simulink model "Tasks_union_3"  (R2020b)
settings: Solver=FixedStepAuto  StartTime=0.0  StopTime=11  FixedStep=0.001  RelTol=1e-3
values from neighbouring files (symbols this model uses):
  a = evalin('base','a')    [Coriolis.m]    (also in init.m = 0.5)
  a0 = 0.99    [init.m]
  ac = mass_can*(l1*l2)    (= 0.5)    [init.m]
  berta = 0.98    [init.m]
  csi = 1    [init.m]
  e_max = 0.01    [init.m]
  F_int_max = [2;2]    [init.m]
  F_max = [2;2]    [init.m]
  g = 9.81    [init.m]
  I1 = evalin('base','I1')    [Mass.m]    (also in init.m = 1)
  I2 = evalin('base','I2')    [Mass.m]    (also in init.m = 1)
  Ic = mass_can*l2^2    (= 0.5)    [init.m]
  k_can = 500    [init.m]
  k_shelf = k_table    (= 10000)    [init.m]
  k_table = 10000    [init.m]
  k_wall = k_table    (= 10000)    [init.m]
  l1 = evalin('base','l1')    [Jacobianoa.m]    (also in Mass.m; cin_dir.m; init.m = 1)
  l2 = evalin('base','l2')    [Jacobianoa.m]    (also in Mass.m; cin_dir.m; init.m = 1)
  l_can = 0.1    [init.m]
  M = 0.1    [init.m]
  m1 = evalin('base','m1')    [Mass.m]    (also in init.m = 1)
  m2 = evalin('base','m2')    [Mass.m]    (also in init.m = 1)
  mass = 0.1    [init.m]
  mass_can = 0.5    [init.m]
  x_can = 0.5    [init.m]
  x_wall = 1.5    [init.m]
  y_shelf = 0.5    [init.m]
  y_table = 0    [init.m]
libraries: simulink x3
settings Model: Creator=chiara-s  LastModifiedBy=giorg

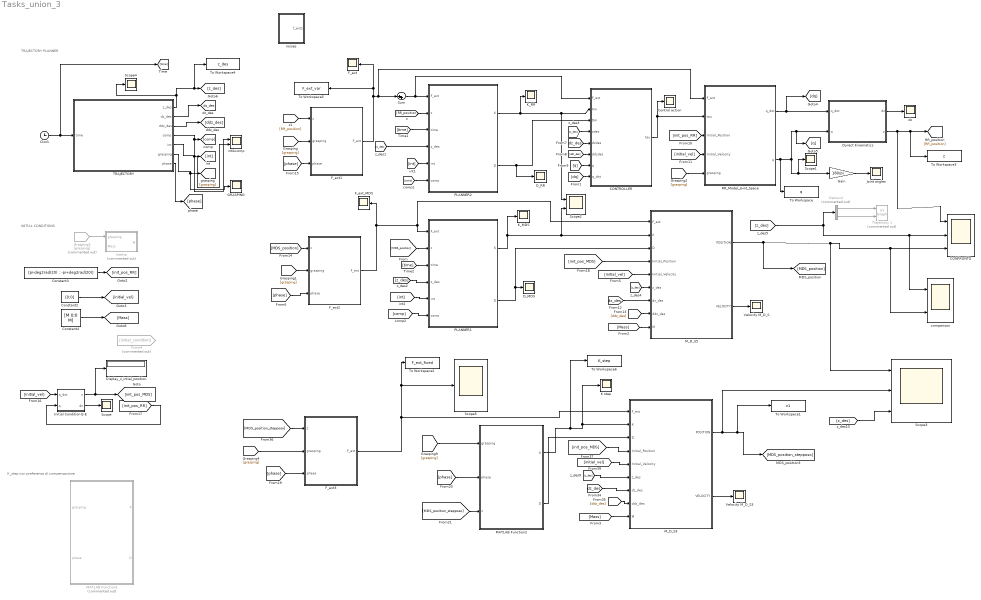
== system Tasks_union_3 ==
  note: K_step con preferenza di compensazione
  note: INITIAL CONDITIONS
  note: TRAJECTORY PLANNER
  CONFRONTO : Scope  NumInputPorts=3
  CONTROLLER : MATLAB Function  TreatAsAtomicUnit=on
  Clock : Clock
  Constant2 : Constant  Value=[0;0]
  Constant3 : Constant  Value=[pi-deg2rad(20) ; -pi+deg2rad(20)]  VectorParams1D=off
  Constant4 : Constant  Value=[M 0;0 M]
  Control action : Scope
  D_MDS : Scope
  D_RR : Scope
  Demux2 : Demux  Commented=on  Outputs=2
  Display_z_intial_position : Display
  Dyrect Kinematics : MATLAB Function  TreatAsAtomicUnit=on
  F_ext : Scope
  F_ext1 : MATLAB Function  TreatAsAtomicUnit=on
  F_ext2 : MATLAB Function  TreatAsAtomicUnit=on
  F_ext3 : MATLAB Function  TreatAsAtomicUnit=on
  F_ext_MDS : Scope
  From4 : From  Commented=on  GotoTag=initial_condition
  GRASPING : Scope
  Gain : Gain  Gain=180/pi
  Grasping3 : From  Commented=on  GotoTag=grasping
  "Inertia " : MATLAB Function  Commented=on  TreatAsAtomicUnit=on
  Initial Condition E-E : MATLAB Function  TreatAsAtomicUnit=on
  Joint angles : Scope
  K step : Scope
  K_MDS : Scope
  K_RR : Scope
  MATLAB Function1 : MATLAB Function  Commented=on  TreatAsAtomicUnit=on
  MATLAB Function2 : MATLAB Function  TreatAsAtomicUnit=on
  M_D_S3 : Subsystem
  M_D_S5 : Subsystem
  PLANNER1 : Subsystem
  PLANNER2 : Subsystem
  RR_Model_Joint_Space : Subsystem
  Scope{,1,4..5} (4 alike) : Scope
  Scope2 : Scope  NumInputPorts=2
  Scope3 : Scope  NumInputPorts=3
  Sum : Sum  Inputs=|++
  TRAJECTORY : Subsystem
  To Workspace : ToWorkspace  VariableName=q  SaveFormat=Timeseries  SampleTime=-1
  To Workspace1 : ToWorkspace  VariableName=z1  SaveFormat=Timeseries  SampleTime=-1
  To Workspace2 : ToWorkspace  VariableName=F_ext_fixed  SaveFormat=Timeseries  SampleTime=-1
  To Workspace3 : ToWorkspace  VariableName=z  SaveFormat=Timeseries  SampleTime=-1
  To Workspace4 : ToWorkspace  VariableName=z_des  SaveFormat=Timeseries  SampleTime=-1
      settings: Save2DSignal=2-D array (concatenate along first dimension)
  To Workspace5 : ToWorkspace  VariableName=F_ext_var  SaveFormat=Timeseries  SampleTime=-1
  To Workspace6 : ToWorkspace  VariableName=K_step  SaveFormat=Timeseries  SampleTime=-1
  Trajectory 1 : simulink/Sinks/XY Graph  Commented=on  xmin=-2  xmax=2  ymin=-2  ymax=2  st=-1
  Velocity M_D_S : Scope
  Velocity M_D_S3 : Scope
  comparison : Scope  NumInputPorts=2
  dz : Scope
  int&comp : Scope  NumInputPorts=2
  noises : Subsystem
  tag scope: dz_des=global
  wires:
  TRAJECTORY/4(comp) -> int&comp/1, [comp]
  [grasping] -> RR_Model_Joint_Space/5(grasping)
  [q] -> CONTROLLER/7(q)
  M_D_S5/1(POSITION) -> [MDS_position], Scope3/1, comparison/2, CONFRONTO/3
  Demux2/1 -> Trajectory 1/1
  M_D_S5/2(VELOCITY) -> Velocity M_D_S/1
  [dz_des] -> CONTROLLER/5(dzdes)
  Initial Condition E-E/2(dz) -> Scope/1
  [ddz_des] -> M_D_S5/8(ddz_des)
  [z_des] -> CONFRONTO/2, comparison/1, Demux2/1
  [grasping] -> F_ext1/2(grasping)
  [initial_vel] -> M_D_S5/5(Initial_Velocity)
  CONTROLLER/1(tau) -> Control action/1, RR_Model_Joint_Space/2(tau)
  [init_pos_RR] -> RR_Model_Joint_Space/3(Initial_Position)
  Gain/1 -> Joint angles/1
  [initial_vel] -> Initial Condition E-E/1(q_dot)
  TRAJECTORY/3(ddz_des) -> [ddz_des]
  RR_Model_Joint_Space/1(q_dot) -> [dq], Dyrect Kinematics/1(q_dot)
  Dyrect Kinematics/1(dz) -> dz/1
  TRAJECTORY/2(dz_des) -> [dz_des]
  Constant4/1 -> [Mass]
  TRAJECTORY/1(z_des) -> [z_des], To Workspace4/1, Scope4/1
  Initial Condition E-E/1(z) -> Display_z_intial_position/1, [init_pos_MDS]
  Constant3/1 -> [init_pos_RR]
  [dz_des] -> M_D_S5/7(dz_des)
  [ddz_des] -> CONTROLLER/6(ddzdes)
  [initial_vel] -> RR_Model_Joint_Space/4(Initial_Velocity)
  F_ext2/1(F_ext) -> PLANNER1/1(F_ext), M_D_S5/1(F_ext), F_ext_MDS/1
  Constant2/1 -> [initial_vel]
  [z_des] -> CONTROLLER/4(zdes)
  TRAJECTORY/6(grasping) -> [grasping], GRASPING/1
  [MDS_position] -> F_ext2/1(z)
  [RR_position] -> F_ext1/1(z)
  Dyrect Kinematics/2(z) -> CONFRONTO/1, To Workspace3/1, [RR_position]
  [grasping] -> F_ext2/2(grasping)
  [z_des] -> M_D_S5/6(z_des)
  Clock/1 -> TRAJECTORY/1(time), [time]
  RR_Model_Joint_Space/2(q) -> To Workspace/1, Scope1/1, Gain/1, Dyrect Kinematics/2(q), [q]
  Grasping3/1 -> "Inertia "/1(grasping)
  [dq] -> CONTROLLER/8(q_dot)
  [init_pos_RR] -> Initial Condition E-E/2(q)
  [Mass] -> M_D_S5/9(M)
  Demux2/2 -> Trajectory 1/2
  TRAJECTORY/5(int) -> int&comp/2, [int]
  TRAJECTORY/7(phase) -> [phase]
  [phase] -> F_ext2/3(phase)
  PLANNER1/1(K) -> K_MDS/1, Scope2/2, M_D_S5/2(K)
  PLANNER1/2(D) -> M_D_S5/3(D), D_MDS/1
  [MDS_position] -> PLANNER1/2(z)
  [time] -> PLANNER1/3(time)
  [z_des] -> PLANNER1/4(z_des)
  [int] -> PLANNER1/5(int)
  [comp] -> PLANNER1/6(comp)
  [phase] -> F_ext1/3(phase)
  F_ext1/1(F_ext) -> RR_Model_Joint_Space/1(F_ext), Sum/1, F_ext/1, To Workspace5/1
  [RR_position] -> PLANNER2/2(z)
  [time] -> PLANNER2/3(time)
  [z_des] -> PLANNER2/4(z_des)
  [comp] -> PLANNER2/6(comp)
  [int] -> PLANNER2/5(int)
  PLANNER2/1(K) -> K_RR/1, Scope2/1, CONTROLLER/2(Km)
  PLANNER2/2(D) -> D_RR/1, CONTROLLER/3(Dm)
  [init_pos_MDS] -> M_D_S5/4(Initial_Position)
  [initial_vel] -> M_D_S3/5(Initial_Velocity)
  MATLAB Function2/2(D) -> M_D_S3/3(D)
  MATLAB Function2/1(K) -> To Workspace6/1, K step/1, M_D_S3/2(K)
  [grasping] -> MATLAB Function2/1(grasping)
  M_D_S3/1(POSITION) -> Scope3/2, To Workspace1/1, [MDS_position_stepposo]
  [init_pos_MDS] -> M_D_S3/4(Initial_Position)
  M_D_S3/2(VELOCITY) -> Velocity M_D_S3/1
  [dz_des] -> M_D_S3/7(dz_des)
  [ddz_des] -> M_D_S3/8(ddz_des)
  [z_des] -> M_D_S3/6(z_des)
  [Mass] -> M_D_S3/9(M)
  [MDS_position_stepposo] -> F_ext3/1(z)
  [grasping] -> F_ext3/2(grasping)
  [phase] -> F_ext3/3(phase)
  F_ext3/1(F_ext) -> M_D_S3/1(F_ext), To Workspace2/1, Scope5/1
  [z_des] -> Scope3/3
  [phase] -> MATLAB Function2/2(phase)
  [MDS_position_stepposo] -> MATLAB Function2/3(z)
  Sum/1 -> CONTROLLER/1(F_ext), PLANNER2/1(F_ext)
  ? -> Sum/2

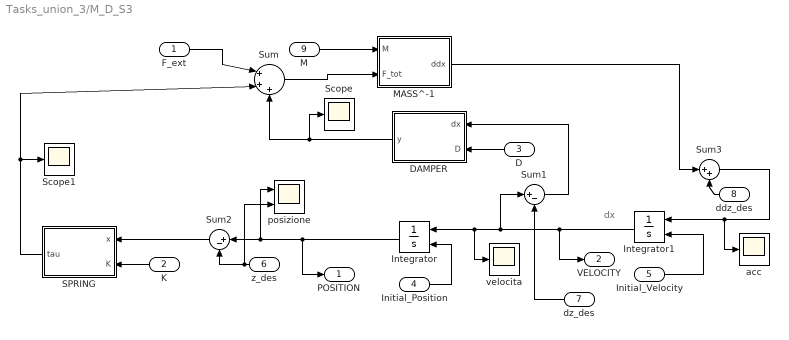
== system Tasks_union_3/M_D_S3 ==
  note: dx
  F_ext : Inport
  K : Inport  Port=2
  D : Inport  Port=3
  Initial_Position : Inport  Port=4
  Initial_Velocity : Inport  Port=5
  z_des : Inport  Port=6
  dz_des : Inport  Port=7
  ddz_des : Inport  Port=8
  M : Inport  Port=9
  DAMPER : MATLAB Function  TreatAsAtomicUnit=on
  Integrator : Integrator  InitialConditionSource=external
  Integrator1 : Integrator  InitialConditionSource=external
  MASS^-1 : MATLAB Function  TreatAsAtomicUnit=on
  SPRING : MATLAB Function  TreatAsAtomicUnit=on
  Scope : Scope
  Scope1 : Scope
  Sum : Sum  Inputs=|+++
  Sum1 : Sum  Inputs=|+-
  Sum2 : Sum  Inputs=|+-
  Sum3 : Sum  Inputs=|++
  acc : Scope
  posizione : Scope  NumInputPorts=2
  velocita : Scope
  POSITION : Outport
  VELOCITY : Outport  Port=2
  wires:
  Integrator1/1 -> velocita/1, Integrator/1, Sum1/1, VELOCITY/1
  SPRING/1(tau) -> Sum/2, Scope1/1
  Integrator/1 -> posizione/1, Sum2/1, POSITION/1
  DAMPER/1(y) -> Scope/1, Sum/3
  Sum/1 -> MASS^-1/2(F_tot)
  M/1 -> MASS^-1/1(M)
  D/1 -> DAMPER/2(D)
  K/1 -> SPRING/2(K)
  Initial_Velocity/1 -> Integrator1/2
  Initial_Position/1 -> Integrator/2
  z_des/1 -> posizione/2, Sum2/2
  Sum2/1 -> SPRING/1(x)
  MASS^-1/1(ddx) -> Sum3/1
  Sum1/1 -> DAMPER/1(dx)
  Sum3/1 -> acc/1, Integrator1/1
  dz_des/1 -> Sum1/2
  ddz_des/1 -> Sum3/2
  F_ext/1 -> Sum/1

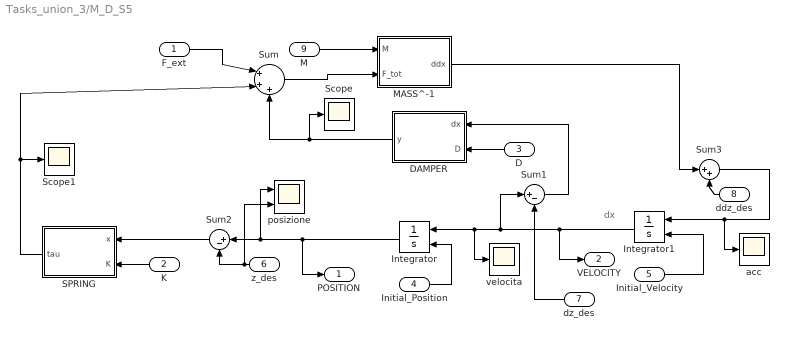
== system Tasks_union_3/M_D_S5 ==
  note: dx
  F_ext : Inport
  K : Inport  Port=2
  D : Inport  Port=3
  Initial_Position : Inport  Port=4
  Initial_Velocity : Inport  Port=5
  z_des : Inport  Port=6
  dz_des : Inport  Port=7
  ddz_des : Inport  Port=8
  M : Inport  Port=9
  DAMPER : MATLAB Function  TreatAsAtomicUnit=on
  Integrator : Integrator  InitialConditionSource=external
  Integrator1 : Integrator  InitialConditionSource=external
  MASS^-1 : MATLAB Function  TreatAsAtomicUnit=on
  SPRING : MATLAB Function  TreatAsAtomicUnit=on
  Scope : Scope
  Scope1 : Scope
  Sum : Sum  Inputs=|+++
  Sum1 : Sum  Inputs=|+-
  Sum2 : Sum  Inputs=|+-
  Sum3 : Sum  Inputs=|++
  acc : Scope
  posizione : Scope  NumInputPorts=2
  velocita : Scope
  POSITION : Outport
  VELOCITY : Outport  Port=2
  wires:
  Integrator1/1 -> velocita/1, Integrator/1, Sum1/1, VELOCITY/1
  SPRING/1(tau) -> Sum/2, Scope1/1
  Integrator/1 -> posizione/1, Sum2/1, POSITION/1
  DAMPER/1(y) -> Scope/1, Sum/3
  Sum/1 -> MASS^-1/2(F_tot)
  M/1 -> MASS^-1/1(M)
  D/1 -> DAMPER/2(D)
  K/1 -> SPRING/2(K)
  Initial_Velocity/1 -> Integrator1/2
  Initial_Position/1 -> Integrator/2
  z_des/1 -> posizione/2, Sum2/2
  Sum2/1 -> SPRING/1(x)
  MASS^-1/1(ddx) -> Sum3/1
  Sum1/1 -> DAMPER/1(dx)
  Sum3/1 -> acc/1, Integrator1/1
  dz_des/1 -> Sum1/2
  ddz_des/1 -> Sum3/2
  F_ext/1 -> Sum/1

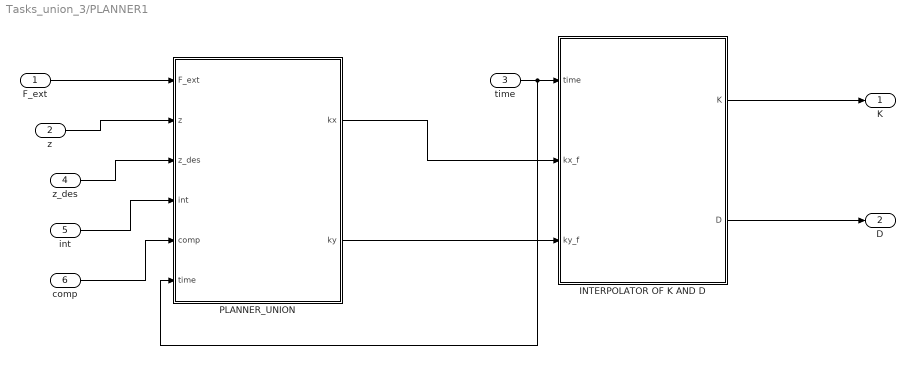
== system Tasks_union_3/PLANNER1 ==
  F_ext : Inport
  z : Inport  Port=2
  time : Inport  Port=3
  z_des : Inport  Port=4
  int : Inport  Port=5
  comp : Inport  Port=6
  "INTERPOLATOR OF K AND D " : MATLAB Function  TreatAsAtomicUnit=on
  PLANNER_UNION : MATLAB Function  TreatAsAtomicUnit=on
  K : Outport
  D : Outport  Port=2
  wires:
  time/1 -> "INTERPOLATOR OF K AND D "/1(time), PLANNER_UNION/6(time)
  "INTERPOLATOR OF K AND D "/2(D) -> D/1
  "INTERPOLATOR OF K AND D "/1(K) -> K/1
  PLANNER_UNION/2(ky) -> "INTERPOLATOR OF K AND D "/3(ky_f)
  PLANNER_UNION/1(kx) -> "INTERPOLATOR OF K AND D "/2(kx_f)
  int/1 -> PLANNER_UNION/4(int)
  comp/1 -> PLANNER_UNION/5(comp)
  F_ext/1 -> PLANNER_UNION/1(F_ext)
  z/1 -> PLANNER_UNION/2(z)
  z_des/1 -> PLANNER_UNION/3(z_des)

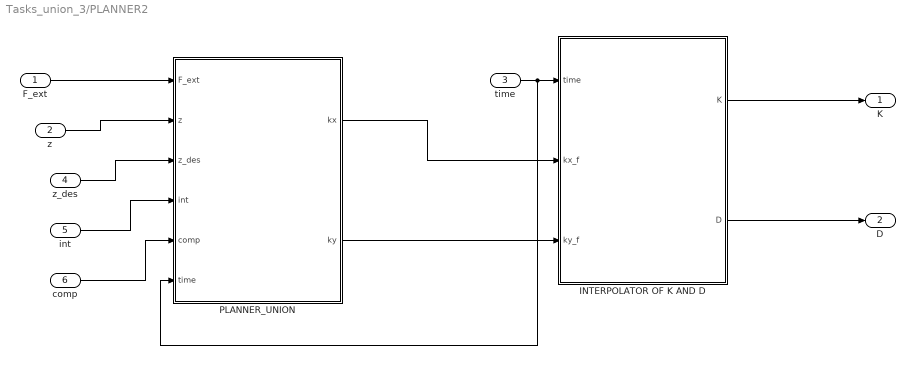
== system Tasks_union_3/PLANNER2 ==
  F_ext : Inport
  z : Inport  Port=2
  time : Inport  Port=3
  z_des : Inport  Port=4
  int : Inport  Port=5
  comp : Inport  Port=6
  "INTERPOLATOR OF K AND D " : MATLAB Function  TreatAsAtomicUnit=on
  PLANNER_UNION : MATLAB Function  TreatAsAtomicUnit=on
  K : Outport
  D : Outport  Port=2
  wires:
  time/1 -> "INTERPOLATOR OF K AND D "/1(time), PLANNER_UNION/6(time)
  "INTERPOLATOR OF K AND D "/2(D) -> D/1
  "INTERPOLATOR OF K AND D "/1(K) -> K/1
  PLANNER_UNION/2(ky) -> "INTERPOLATOR OF K AND D "/3(ky_f)
  PLANNER_UNION/1(kx) -> "INTERPOLATOR OF K AND D "/2(kx_f)
  int/1 -> PLANNER_UNION/4(int)
  comp/1 -> PLANNER_UNION/5(comp)
  F_ext/1 -> PLANNER_UNION/1(F_ext)
  z/1 -> PLANNER_UNION/2(z)
  z_des/1 -> PLANNER_UNION/3(z_des)

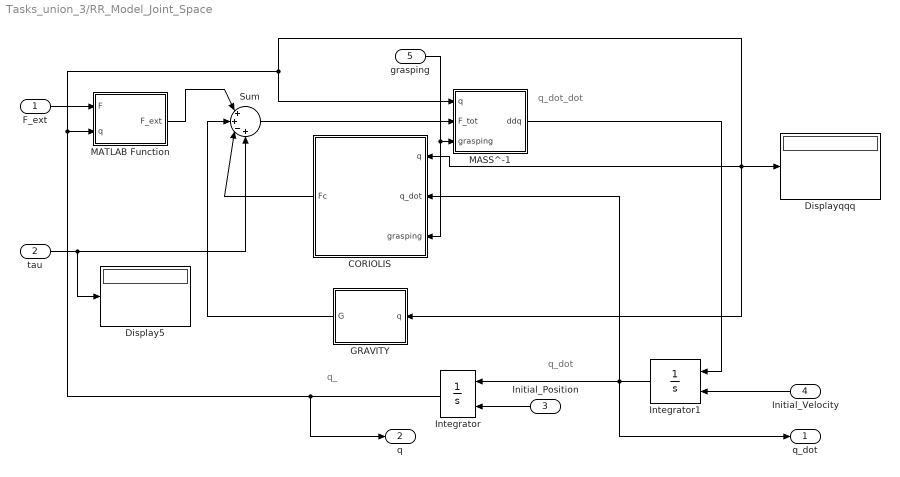
== system Tasks_union_3/RR_Model_Joint_Space ==
  note: q_dot
  note: q_dot_dot
  note: q_
  F_ext : Inport
  tau : Inport  Port=2
  Initial_Position : Inport  Port=3
  Initial_Velocity : Inport  Port=4
  grasping : Inport  Port=5
  CORIOLIS : MATLAB Function  TreatAsAtomicUnit=on
  Display5 : Display
  Displayqqq : Display
  GRAVITY : MATLAB Function  TreatAsAtomicUnit=on
  Integrator : Integrator  InitialConditionSource=external
  Integrator1 : Integrator  InitialConditionSource=external  InitialCondition=[0;0]
  MASS^-1 : MATLAB Function  TreatAsAtomicUnit=on
  MATLAB Function : MATLAB Function  TreatAsAtomicUnit=on
  Sum : Sum  Inputs=|++-+
  q_dot : Outport
  q : Outport  Port=2
  wires:
  GRAVITY/1(G) -> Sum/2
  MATLAB Function/1(F_ext) -> Sum/1
  Initial_Position/1 -> Integrator/2
  F_ext/1 -> MATLAB Function/1(F)
  Integrator/1 -> MASS^-1/1(q), GRAVITY/1(q), Displayqqq/1, CORIOLIS/1(q), MATLAB Function/2(q), q/1
  Integrator1/1 -> q_dot/1, CORIOLIS/2(q_dot), Integrator/1
  Initial_Velocity/1 -> Integrator1/2
  MASS^-1/1(ddq) -> Integrator1/1
  Sum/1 -> MASS^-1/2(F_tot)
  CORIOLIS/1(Fc) -> Sum/3
  tau/1 -> Display5/1, Sum/4
  grasping/1 -> CORIOLIS/3(grasping), MASS^-1/3(grasping)

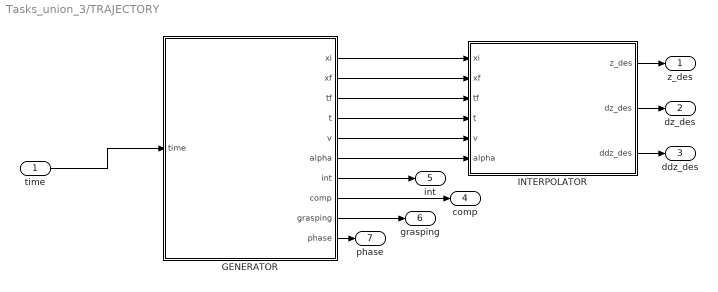
== system Tasks_union_3/TRAJECTORY ==
  time : Inport
  GENERATOR : MATLAB Function  TreatAsAtomicUnit=on
  INTERPOLATOR : MATLAB Function  TreatAsAtomicUnit=on
  z_des : Outport
  dz_des : Outport  Port=2
  ddz_des : Outport  Port=3
  comp : Outport  Port=4
  int : Outport  Port=5
  grasping : Outport  Port=6
  phase : Outport  Port=7
  wires:
  GENERATOR/1(xi) -> INTERPOLATOR/1(xi)
  GENERATOR/2(xf) -> INTERPOLATOR/2(xf)
  GENERATOR/3(tf) -> INTERPOLATOR/3(tf)
  GENERATOR/4(t) -> INTERPOLATOR/4(t)
  GENERATOR/5(v) -> INTERPOLATOR/5(v)
  GENERATOR/6(alpha) -> INTERPOLATOR/6(alpha)
  INTERPOLATOR/1(z_des) -> z_des/1
  INTERPOLATOR/2(dz_des) -> dz_des/1
  INTERPOLATOR/3(ddz_des) -> ddz_des/1
  GENERATOR/7(int) -> int/1
  GENERATOR/8(comp) -> comp/1
  GENERATOR/9(grasping) -> grasping/1
  GENERATOR/10(phase) -> phase/1
  time/1 -> GENERATOR/1(time)

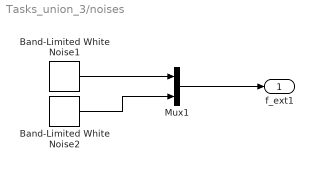
== system Tasks_union_3/noises ==
  Band-Limited White Noise1 : simulink/Sources/Band-Limited White Noise  Cov=0.0001  Ts=0.001  seed=[randi(10000,1)]
  Band-Limited White Noise2 : simulink/Sources/Band-Limited White Noise  Cov=0.0001  Ts=0.001  seed=[randi(10000,1)]
  Mux1 : Mux  Inputs=2
  f_ext1 : Outport
  wires:
  Band-Limited White Noise2/1 -> Mux1/2
  Band-Limited White Noise1/1 -> Mux1/1
  Mux1/1 -> f_ext1/1

== matlab function Tasks_union_3/Dyrect Kinematics ==
  data: q_dot input double size=2; dz output double size=2; q input double size=2; z output double size=2; l1 parameter; l2 parameter
function [dz,z] = fcn(q_dot,q,l1, l2)

z = zeros(2,1);
z(1) = l1*cos(q(1)) + l2*cos(q(1)+q(2));
z(2) = l1*sin(q(1)) + l2*sin(q(1)+q(2));

Ja = zeros(2,2);
Ja = [-l1*sin(q(1)) - l2*sin(q(1)+q(2)), -l2*sin(q(1)+q(2)); ...
    l1*cos(q(1)) + l2*cos(q(1)+q(2)), l2*cos(q(1)+q(2))];

dz = zeros(2,1);
dz = Ja*q_dot;

end

== matlab function Tasks_union_3/PLANNER1/INTERPOLATOR OF K AND D  ==
  settings: updateMethod=DISCRETE  sampleTime=Ts
  data: time input; K output; kx_f input; ky_f input; D output; e_max parameter; F_max parameter; M parameter; berta parameter; a0 parameter; mass parameter; csi parameter
function [K,D] = fcn(time, kx_f, ky_f, e_max, F_max,M, berta, a0, mass, csi)

persistent kx ky time_prec

if isempty(time_prec)
    time_prec = 0;
end

if isempty(kx)
   kx = F_max(1)/e_max; 
end
if isempty(ky)
   ky = F_max(2)/e_max;
end

% everytime k is increasing in accordance with stability condition
if kx_f <= kx
    kx = kx_f;
else 
    kx_i = kx;
    k_dotx = berta*(4*a0*sqrt(kx_i/mass)*(kx_i)^(3/2))/(sqrt(kx_i) + 2*a0*csi*sqrt(kx_i));
    k_tempx = kx_i + k_dotx*(time -time_prec);
    if k_tempx > kx_f
        kx = kx_f;
    else
        kx = k_tempx;
    end
end

if ky_f <= ky
    ky = ky_f;
else 
    ky_i = ky;
    k_doty = berta*(4*a0*sqrt(ky_i/mass)*(ky_i)^(3/2))/(sqrt(ky_i) + 2*a0*csi*sqrt(ky_i));
    k_tempy = ky_i + k_doty*(time -time_prec);
    if k_tempy > ky_f
        ky = ky_f;
    else
        ky = k_tempy;
    end
end
time_prec = time;

dx = sqrt(4*kx*M);
dy = sqrt(4*ky*M);

D = diag([dx,dy]);
K = diag([kx,ky]);

end

== matlab function Tasks_union_3/F_ext3 ==
  data: z input; F_ext output; grasping input; mass_can parameter; g parameter; phase input; x_can parameter; y_table parameter; k_can parameter; k_table parameter; l_can parameter; x_wall parameter; y_shelf parameter; k_wall parameter; k_shelf parameter
function F_ext = fcn(z, grasping, mass_can, g, phase, x_can, y_table, k_can, k_table, l_can, x_wall, y_shelf, k_wall, k_shelf) 

% hypothesis: table reaction force with elastic behaviour
F_ext = zeros(2,1);

if phase == 1
    % if contact is happened with can
    if grasping == 0
        if z(1) > x_can
            F_ext(1) = -k_can*(z(1) - x_can);    
        end
        if z(2) < y_table
            F_ext(2) = -k_table*(z(2) - y_table);
        end
    else 
        if z(2) < y_table
            F_ext(2) = -k_table*(z(2)-y_table);       
        else 
            if (abs(k_table*(z(2)-y_table)) < abs(mass_can*g))
                F_ext(2) = - k_table*(z(2)-y_table); 
            else 
                F_ext(2) = - mass_can*g;
            end    
        end
    end
elseif phase == 2
    if z(1) + l_can > x_wall 
        F_ext(1) = -k_wall*(z(1) + l_can -x_wall);
    end
    if z(2) < y_shelf
        F_ext(2) = -k_shelf*(z(2) - y_shelf);
    else 
        if (abs(k_shelf*(z(2)-y_shelf)) < abs(mass_can*g))
            F_ext(2) = - k_shelf*(z(2)-y_shelf); 
        else 
            F_ext(2) = - mass_can*g;
        end 
    end
else
    if z(1) + l_can > x_wall 
        F_ext(1) = -k_wall*(z(1) + l_can -x_wall);
    end
    if z(2) < y_shelf
        F_ext(2) = -k_shelf*(z(2) - y_shelf);
    end
end

== matlab function Tasks_union_3/MATLAB Function1 ==
  data: grasping input; phase input; K output; D output; M parameter
function [K,D] = fcn(grasping,phase,M)
k1 = 200;
k2 = 200;
if phase == 1
    if grasping == 0
      k1 = 20;
      k2 = 20;
    else
      k1 = 200;
      k2 = 490.5; 
    end
elseif phase == 2 
     k1 = 20;
     k2 = 490.5;
elseif phase == 3
     k1 = 20;
     k2 = 20;
end
K = [k1 0; 0 k2];
D = [sqrt(4*M*k1) 0; 0 sqrt(4*M*k2)];
end

== matlab function Tasks_union_3/PLANNER1/PLANNER_UNION ==
  settings: updateMethod=DISCRETE  sampleTime=Ts
  data: kx output; F_ext input; z input; z_des input; int input; comp input; ky output; e_max parameter; F_max parameter; F_int_max parameter; time input
function [kx, ky] = fcn(F_ext, z, z_des, int, comp, e_max, F_max, F_int_max, time)
%% Description MDS_interaction


%% Outputs
% K            stiffness 
% D            damping 

%% Inputs
% time          current simulation time
% F_ext         measured external force
% mass          mass scalar value 
% F_int_max     desired interaction force
% z_des         desired trajectory
% z             current position
% F_max         estimated force disturbances
% e_max         maximum steady-state error

persistent kxi kyi kxc kyc F_comp
persistent int_prec comp_prec z_int z_int_dir 

% persistent initialization
if isempty(kxi)
   kxi = F_max(1)/e_max; 
end
if isempty(F_comp)
   F_comp = [0;0];
end

if isempty(kyi)
   kyi = F_max(2)/e_max;
end
if isempty(kxc)
      kxc = F_max(1)/e_max;
end
if isempty(kyc)
      kyc = F_max(2)/e_max;
end
if isempty(z_int) 
    z_int = [1000; 1000];
end
if isempty(z_int_dir) 
    z_int_dir = [0;0];
end
if isempty(int_prec)
    int_prec = [0;0];
end
if isempty(comp_prec)
    comp_prec = [0;0];
end

% interaction X axes
if int(1) == 1
    if abs(F_ext(1)-F_comp(1)) > F_max(1)         % F_max soglia dei disturbi
        if z_int(1) == 1000
            z_int(1) = z(1);
            z_int_dir(1) = -sign(F_ext(1)-F_comp(1));     % direzione non permessa
        end
    end
    if abs(F_ext(1)-F_comp(1)) > F_int_max(1) 
            % if interaction force is higher than threshold
            if kxi*abs(z(1)-z_des(1)) > F_int_max(1)
                % set k 
                ktemp_x = F_int_max(1)/abs(z(1)-z_des(1));
                if ktemp_x < kxi
                    kxi = ktemp_x;
                end
            end
    end
end

% interaction Y axes
if int(2) == 1
    if abs(F_ext(2)-F_comp(2)) > F_max(2)         % F_max soglia dei disturbi
        if z_int(2) == 1000
            z_int(2) = z(2);
            z_int_dir(2) = -sign(F_ext(2)-F_comp(2));     % direzione non permessa
        end
    end
    % Similarly for the other direction
    if abs(F_ext(2)-F_comp(2)) > F_int_max(2) 
            if kyi*abs(z(2)-z_des(2)) > F_int_max(2)
                ktemp_y = F_int_max(2)/abs(z(2)-z_des(2));
                if ktemp_y < kyi
                    kyi = ktemp_y;
                end
            end
    end
end

% compensation X axes
if comp(1) == 1
    if z_int(1) == 1000
       if abs(F_ext(1))/kxc > e_max
            kxc = abs(F_ext(1))/e_max;
            F_comp(1) = F_ext(1);
       end
    else 
        if z_int_dir(1) == 1
            if z(1) < z_int(1)
                if abs(F_ext(1))/kxc > e_max 
                    kxc = abs(F_ext(1))/e_max;
                    F_comp(1) = F_ext(1);
                end
            end
        else
            if z(1) > z_int(1)
                if abs(F_ext(1))/kxc > e_max
                    kxc = abs(F_ext(1))/e_max;
                    F_comp(1) = F_ext(1);
                end
            end
        end
                
   end
end

% compensation Y axes
if comp(2) == 1
    if z_int(2) == 1000 
       if abs(F_ext(2))/kyc > e_max
            kyc = abs(F_ext(2))/e_max;
            F_comp(2) = F_ext(2);
       end
    else 
        if z_int_dir(2) == 1
            if z(2) < z_int(2)
                if abs(F_ext(2))/kyc > e_max
                    kyc = abs(F_ext(2))/e_max;
                    F_comp(2) = F_ext(2);
                end
            end
        else
            if z(2) > z_int(2)
                if abs(F_ext(2))/kyc > e_max
                    kyc = abs(F_ext(2))/e_max;
                    F_comp(2) = F_ext(2);
                end
            end
        end
                
   end
end

% reset to default
if comp(1)==0 && comp_prec(1)==1
%     z_int_dir(1) = 0;
%     z_int(1) = 1000;
    kxc = F_max(1)/e_max;
    F_comp(1) = 0;
end
if comp(2)==0 && comp_prec(2)==1
%     z_int_dir(2) = 0;
%     z_int(2) = 1000;
    kyc = F_max(2)/e_max;
    F_comp(2) = 0;
end
if int(1)==0 && int_prec(1)==1
    kxi = F_max(1)/e_max;
end
if int(2)==0 && int_prec(2)==1
    kyi = F_max(2)/e_max;
end
% quando c'è una interazione e prima non c'era risetto tutto (RACCAPEZZO)
if int(1)==1 && int_prec(1)==0
    if comp_prec(1) == 1
        kxi = kxc;
    end
    z_int(1)=1000;
    z_int_dir(1)=0;
end
if int(2)==1 && int_prec(2)==0
    if comp_prec(2) == 1
        kyi = kyc;
    end
    z_int(2)=1000;
    z_int_dir(2)=0;
end
if comp(1) == 1 && comp_prec(1)==0
    if int_prec(1) == 1
        kxc = kxi;
    end
end
if comp(2) == 1 && comp_prec(2)==0
    if int_prec(2)==1
        kyc =kyi;
    end
end
% update last booleans
int_prec = int;
comp_prec = comp;


% Final Values of D-K
kx = abs(F_max(1))/e_max;
ky = abs(F_max(2))/e_max;

if comp(1) == 1
    kx = kxc;
end
if comp(2) == 1
    ky = kyc;
end
if int(1) == 1
    kx = kxi;
    if comp(1) == 1
        if z_int(1) == 1000
            kx = kxc;
        else
            if z_int_dir(1) == 1
                if z_des(1) < z_int(1)
                    kx = kxc;
                end
            else
                if z_des(1) > z_int(1)
                    kx = kxc;
                end
            end
        end
    else
        if z_int(1) == 1000
            kx = F_max(1)/e_max;
        else
            if z_int_dir(1) == 1
                if z_des(1) < z_int(1)
                    kx = F_max(1)/e_max;
                end
            else
                if z_des(1) > z_int(1)
                    kx = F_max(1)/e_max;
                end
            end
        end
    end
end
if int(2) == 1
    ky = kyi;
     if comp(2) == 1
        if z_int(2) == 1000
            kx = kxc;
        else
            if z_int_dir(2) == 1
                if z_des(2) < z_int(2) 
                    ky = kyc;
                end
            else
                if z_des(2) > z_int(2)
                    ky = kyc;
                end
            end
        end
     else
         if z_int(2) == 1000
            kx = F_max(2)/e_max;
        else
            if z_int_dir(2) == 1
                if z_des(2) < z_int(2) 
                    ky = F_max(2)/e_max;
                end
            else
                if z_des(2) > z_int(2)
                    ky = F_max(2)/e_max;
                end
            end
        end
     end
end

end

== matlab function Tasks_union_3/TRAJECTORY/GENERATOR ==
  data: time input; xi output; xf output; tf output; t output; v output; alpha output; int output; comp output; grasping output; phase output
function  [xi, xf, tf, t, v, alpha, int, comp, grasping, phase] = fcn(time)

alpha = 0.1;
phase = 1;
int = [1; 1];
comp = [0; 0];
grasping = 0;

if time >= 0 && time < 2
    tf = 2;
    xi = [0; 0.3];
    xf = [0.7; -0.1];
    v = [(xf(1) - xi(1))/((1-alpha)*tf); (xf(2) - xi(2))/((1-alpha)*tf)];
    t = time;
elseif time >= 2 && time < 3
    tf = 1;
    xf = [0.7; -0.1];
    xi = xf; 
    v = [(xf(1) - xi(1))/((1-alpha)*tf); (xf(2) - xi(2))/((1-alpha)*tf)];
    t = time - 2;
elseif time >= 3 && time < 5
    tf = 2;
    xf = [0.7; 1];
    xi = [0.7; -0.1];
    v = [(xf(1) - xi(1))/((1-alpha)*tf); (xf(2) - xi(2))/((1-alpha)*tf)];
    t = time - 3;
    grasping = 1; 
    int = [0; 1];
    comp = [0; 1];
    if time > 4.7
        int = [0; 0];
    end
elseif time >= 5 && time < 7
    tf = 2; 
    xf = [1.6; 0.4];
    xi = [0.7; 1];
    v = [(xf(1) - xi(1))/((1-alpha)*tf); (xf(2) - xi(2))/((1-alpha)*tf)];
    t = time - 5;
    phase = 2; 
    grasping = 1;
    int = [1; 1];
    comp = [0; 1];
elseif time >= 7 && time < 10
    tf = 3;
    xf = [0.7; 1];
    xi = [1.6; 0.4];
    v = [(xf(1) - xi(1))/((1-alpha)*tf); (xf(2) - xi(2))/((1-alpha)*tf)]; 
    t = time - 7; 
    phase = 3; 
    grasping = 0; 
    int = [1; 1];
    comp = [0; 0];
else 
    tf = 1000;
    xf = [0.7; 1];
    xi = xf; 
    v = [(xf(1) - xi(1))/((1-alpha)*tf); (xf(2) - xi(2))/((1-alpha)*tf)]; 
    t = time - 10; 
    phase = 3; 
    grasping = 0; 
    int = [0; 0];
    comp =[0; 0];
end































% if time >= 0 && time < 1
%     tf = 1;
%     xi = [0; 0.3];
%     xf = [0.7; -0.1];
%     v = [(xf(1) - xi(1))/((1-alpha)*tf); (xf(2) - xi(2))/((1-alpha)*tf)];
%     t = time;
% elseif time >= 1 && time < 2
%     tf = 1;
%     xf = [0.7; -0.1];
%     xi = xf; 
%     v = [(xf(1) - xi(1))/((1-alpha)*tf); (xf(2) - xi(2))/((1-alpha)*tf)];
%     t = time - 1;
% elseif time >= 2 && time < 2.5
%     tf = 0.5;
%     xf = [0.7; 1];
%     xi = [0.7; -0.1];
%     v = [(xf(1) - xi(1))/((1-alpha)*tf); (xf(2) - xi(2))/((1-alpha)*tf)];
%     t = time - 2;
%     grasping = 1; 
%     int = [0; 1];
%     comp = [0; 1];
%     if time > 2.49
%         int = [0; 0];
%     end
% elseif time >= 2.5 && time < 3.5
%     tf = 1; 
%     xf = [1.6; 0.4];
%     xi = [0.7; 1];
%     v = [(xf(1) - xi(1))/((1-alpha)*tf); (xf(2) - xi(2))/((1-alpha)*tf)];
%     t = time - 2.5;
%     phase = 2; 
%     grasping = 1;
%     int = [1; 1];
%     comp = [0; 1];
% elseif time >= 3.5 && time < 5
%     tf = 1.5;
%     xf = [0.7; 1];
%     xi = [1.6; 0.4];
%     v = [(xf(1) - xi(1))/((1-alpha)*tf); (xf(2) - xi(2))/((1-alpha)*tf)]; 
%     t = time - 3.5; 
%     phase = 3; 
%     grasping = 0; 
%     int = [1; 1];
%     comp = [0; 0];
% else 
%     tf = 1000;
%     xf = [0.7; 1];
%     xi = xf; 
%     v = [(xf(1) - xi(1))/((1-alpha)*tf); (xf(2) - xi(2))/((1-alpha)*tf)]; 
%     t = time - 5; 
%     phase = 3; 
%     grasping = 0; 
%     int = [0; 0];
%     comp =[0; 0];
% end

end

== matlab function Tasks_union_3/Inertia  ==
  data: M output; grasping input; mass_can parameter; Mass input
function M = fcn(grasping, mass_can, Mass)

if grasping == 1
    M = diag([Mass(1,1)+mass_can Mass(2,2)+mass_can]);
else
    M = Mass;
end

end

== matlab function Tasks_union_3/CONTROLLER ==
  data: F_ext input; Km input; Dm input; zdes input size=2; tau output double size=2; dzdes input size=2; ddzdes input size=2; q input size=2; q_dot input size=2; M parameter
function tau = fcn(F_ext,Km, Dm,zdes, dzdes, ddzdes, q, q_dot, M)
%% PROBLEMA MATRICE DELLE MASSE NON DIAGONALE
coder.extrinsic('Jacobianoa','Jacobianoa_dot','Mass','Coriolis','Gravity','cin_dir')
dz = zeros(2,1);
z = zeros(2,1);
B = zeros(2,2);
S = zeros(2,2);
G = zeros(2,1);
Ja = zeros(2,2);
Ja_dot = zeros(2,2);
Bm = [M 0; 0 M];
Ja = Jacobianoa(q);
Ja_dot = Jacobianoa_dot(q,q_dot);

dz = Ja*q_dot;
z = cin_dir(q);

t = 0.1;
if (deg2rad(-0.1) < q(2)) && (q(2) < deg2rad(0.1)) || (deg2rad(179.9) < q(2)) && (q(2) < deg2rad(180.1)) || (deg2rad(-180.1) < q(2)) && (q(2) < deg2rad(-179.9))
    Ja_inv = (Ja')*inv(Ja*(Ja') + t^2*eye(2,2)); % Damp least square Jacobian method
else 
    Ja_inv = inv(Ja);
end

% Ja_inv = inv(Ja);

B = Mass(q);
Bx = (Ja_inv')* B * Ja_inv;
S = Coriolis(q,q_dot);
G = Gravity(q);
I = eye(2,2);
% tau = B * Ja_inv*(ddzdes - Ja_dot*q_dot) + ...
%     S*q_dot + (Ja')*(Dm*(dzdes - dz) + Km*(zdes- z)) + G;

tau = B*Ja_inv*(ddzdes - Ja_dot*q_dot + ...
    inv(Bm)*(Dm*(dzdes - dz) + Km*(zdes- z))) + S*q_dot - G + ...
    (Ja')*(Bx*inv(Bm) - I)*F_ext;

end

== matlab function Tasks_union_3/Initial Condition E-E ==
  data: q_dot input double size=2; q input double size=2; z output double size=2; dz output double size=2; l1 parameter; l2 parameter
function [z,dz] = fcn(q_dot,q,l1, l2)

z = zeros(2,1);
z(1) = l1*cos(q(1)) + l2*cos(q(1)+q(2));
z(2) = l1*sin(q(1)) + l2*sin(q(1)+q(2));

Ja = zeros(2,2);
Ja = [-l1*sin(q(1)) - l2*sin(q(1)+q(2)), -l2*sin(q(1)+q(2)); ...
    l1*cos(q(1)) + l2*cos(q(1)+q(2)), l2*cos(q(1)+q(2))];

dz = zeros(2,1);
dz = Ja*q_dot;

end

== matlab function Tasks_union_3/PLANNER2/INTERPOLATOR OF K AND D  ==
  settings: updateMethod=DISCRETE  sampleTime=Ts
  data: time input; K output; kx_f input; ky_f input; D output; e_max parameter; F_max parameter; M parameter; berta parameter; a0 parameter; mass parameter; csi parameter
function [K,D] = fcn(time, kx_f, ky_f, e_max, F_max,M, berta, a0, mass, csi)

persistent kx ky time_prec

if isempty(time_prec)
    time_prec = 0;
end

if isempty(kx)
   kx = F_max(1)/e_max; 
end
if isempty(ky)
   ky = F_max(2)/e_max;
end

% everytime k is increasing in accordance with stability condition
if kx_f <= kx
    kx = kx_f;
else 
    kx_i = kx;
    k_dotx = berta*(4*a0*sqrt(kx_i/mass)*(kx_i)^(3/2))/(sqrt(kx_i) + 2*a0*csi*sqrt(kx_i));
    k_tempx = kx_i + k_dotx*(time -time_prec);
    if k_tempx > kx_f
        kx = kx_f;
    else
        kx = k_tempx;
    end
end

if ky_f <= ky
    ky = ky_f;
else 
    ky_i = ky;
    k_doty = berta*(4*a0*sqrt(ky_i/mass)*(ky_i)^(3/2))/(sqrt(ky_i) + 2*a0*csi*sqrt(ky_i));
    k_tempy = ky_i + k_doty*(time -time_prec);
    if k_tempy > ky_f
        ky = ky_f;
    else
        ky = k_tempy;
    end
end
time_prec = time;

dx = sqrt(4*kx*M);
dy = sqrt(4*ky*M);

D = diag([dx,dy]);
K = diag([kx,ky]);

end

== matlab function Tasks_union_3/PLANNER2/PLANNER_UNION ==
  settings: updateMethod=DISCRETE  sampleTime=Ts
  data: kx output; F_ext input; z input; z_des input; int input; comp input; ky output; e_max parameter; F_max parameter; F_int_max parameter; time input
function [kx, ky] = fcn(F_ext, z, z_des, int, comp, e_max, F_max, F_int_max, time)
%% Description MDS_interaction


%% Outputs
% K            stiffness 
% D            damping 

%% Inputs
% time          current simulation time
% F_ext         measured external force
% mass          mass scalar value 
% F_int_max     desired interaction force
% z_des         desired trajectory
% z             current position
% F_max         estimated force disturbances
% e_max         maximum steady-state error

persistent kxi kyi kxc kyc F_comp
persistent int_prec comp_prec z_int z_int_dir 

% persistent initialization
if isempty(kxi)
   kxi = F_max(1)/e_max; 
end
if isempty(F_comp)
   F_comp = [0;0];
end

if isempty(kyi)
   kyi = F_max(2)/e_max;
end
if isempty(kxc)
      kxc = F_max(1)/e_max;
end
if isempty(kyc)
      kyc = F_max(2)/e_max;
end
if isempty(z_int) 
    z_int = [1000; 1000];
end
if isempty(z_int_dir) 
    z_int_dir = [0;0];
end
if isempty(int_prec)
    int_prec = [0;0];
end
if isempty(comp_prec)
    comp_prec = [0;0];
end

% interaction X axes
if int(1) == 1
    if abs(F_ext(1)-F_comp(1)) > F_max(1)         % F_max soglia dei disturbi
        if z_int(1) == 1000
            z_int(1) = z(1);
            z_int_dir(1) = -sign(F_ext(1)-F_comp(1));     % direzione non permessa
        end
    end
    if abs(F_ext(1)-F_comp(1)) > F_int_max(1) 
            % if interaction force is higher than threshold
            if kxi*abs(z(1)-z_des(1)) > F_int_max(1)
                % set k 
                ktemp_x = F_int_max(1)/abs(z(1)-z_des(1));
                if ktemp_x < kxi
                    kxi = ktemp_x;
                end
            end
    end
end

% interaction Y axes
if int(2) == 1
    if abs(F_ext(2)-F_comp(2)) > F_max(2)         % F_max soglia dei disturbi
        if z_int(2) == 1000
            z_int(2) = z(2);
            z_int_dir(2) = -sign(F_ext(2)-F_comp(2));     % direzione non permessa
        end
    end
    % Similarly for the other direction
    if abs(F_ext(2)-F_comp(2)) > F_int_max(2) 
            if kyi*abs(z(2)-z_des(2)) > F_int_max(2)
                ktemp_y = F_int_max(2)/abs(z(2)-z_des(2));
                if ktemp_y < kyi
                    kyi = ktemp_y;
                end
            end
    end
end

% compensation X axes
if comp(1) == 1
    if z_int(1) == 1000
       if abs(F_ext(1))/kxc > e_max
            kxc = abs(F_ext(1))/e_max;
            F_comp(1) = F_ext(1);
       end
    else 
        if z_int_dir(1) == 1
            if z(1) < z_int(1)
                if abs(F_ext(1))/kxc > e_max 
                    kxc = abs(F_ext(1))/e_max;
                    F_comp(1) = F_ext(1);
                end
            end
        else
            if z(1) > z_int(1)
                if abs(F_ext(1))/kxc > e_max
                    kxc = abs(F_ext(1))/e_max;
                    F_comp(1) = F_ext(1);
                end
            end
        end
                
   end
end

% compensation Y axes
if comp(2) == 1
    if z_int(2) == 1000 
       if abs(F_ext(2))/kyc > e_max
            kyc = abs(F_ext(2))/e_max;
            F_comp(2) = F_ext(2);
       end
    else 
        if z_int_dir(2) == 1
            if z(2) < z_int(2)
                if abs(F_ext(2))/kyc > e_max
                    kyc = abs(F_ext(2))/e_max;
                    F_comp(2) = F_ext(2);
                end
            end
        else
            if z(2) > z_int(2)
                if abs(F_ext(2))/kyc > e_max
                    kyc = abs(F_ext(2))/e_max;
                    F_comp(2) = F_ext(2);
                end
            end
        end
                
   end
end

% reset to default
if comp(1)==0 && comp_prec(1)==1
%     z_int_dir(1) = 0;
%     z_int(1) = 1000;
    kxc = F_max(1)/e_max;
    F_comp(1) = 0;
end
if comp(2)==0 && comp_prec(2)==1
%     z_int_dir(2) = 0;
%     z_int(2) = 1000;
    kyc = F_max(2)/e_max;
    F_comp(2) = 0;
end
if int(1)==0 && int_prec(1)==1
    kxi = F_max(1)/e_max;
end
if int(2)==0 && int_prec(2)==1
    kyi = F_max(2)/e_max;
end
% quando c'è una interazione e prima non c'era risetto tutto (RACCAPEZZO)
if int(1)==1 && int_prec(1)==0
    if comp_prec(1) == 1
        kxi = kxc;
    end
    z_int(1)=1000;
    z_int_dir(1)=0;
end
if int(2)==1 && int_prec(2)==0
    if comp_prec(2) == 1
        kyi = kyc;
    end
    z_int(2)=1000;
    z_int_dir(2)=0;
end
if comp(1) == 1 && comp_prec(1)==0
    if int_prec(1) == 1
        kxc = kxi;
    end
end
if comp(2) == 1 && comp_prec(2)==0
    if int_prec(2)==1
        kyc =kyi;
    end
end
% update last booleans
int_prec = int;
comp_prec = comp;


% Final Values of D-K
kx = abs(F_max(1))/e_max;
ky = abs(F_max(2))/e_max;

if comp(1) == 1
    kx = kxc;
end
if comp(2) == 1
    ky = kyc;
end
if int(1) == 1
    kx = kxi;
    if comp(1) == 1
        if z_int(1) == 1000
            kx = kxc;
        else
            if z_int_dir(1) == 1
                if z_des(1) < z_int(1)
                    kx = kxc;
                end
            else
                if z_des(1) > z_int(1)
                    kx = kxc;
                end
            end
        end
    else
        if z_int(1) == 1000
            kx = F_max(1)/e_max;
        else
            if z_int_dir(1) == 1
                if z_des(1) < z_int(1)
                    kx = F_max(1)/e_max;
                end
            else
                if z_des(1) > z_int(1)
                    kx = F_max(1)/e_max;
                end
            end
        end
    end
end
if int(2) == 1
    ky = kyi;
     if comp(2) == 1
        if z_int(2) == 1000
            kx = kxc;
        else
            if z_int_dir(2) == 1
                if z_des(2) < z_int(2) 
                    ky = kyc;
                end
            else
                if z_des(2) > z_int(2)
                    ky = kyc;
                end
            end
        end
     else
         if z_int(2) == 1000
            kx = F_max(2)/e_max;
        else
            if z_int_dir(2) == 1
                if z_des(2) < z_int(2) 
                    ky = F_max(2)/e_max;
                end
            else
                if z_des(2) > z_int(2)
                    ky = F_max(2)/e_max;
                end
            end
        end
     end
end

end

== matlab function Tasks_union_3/F_ext2 ==
  data: z input; F_ext output; grasping input; mass_can parameter; g parameter; phase input; x_can parameter; y_table parameter; k_can parameter; k_table parameter; l_can parameter; x_wall parameter; y_shelf parameter; k_wall parameter; k_shelf parameter
function F_ext = fcn(z, grasping, mass_can, g, phase, x_can, y_table, k_can, k_table, l_can, x_wall, y_shelf, k_wall, k_shelf) 

% hypothesis: table reaction force with elastic behaviour
F_ext = zeros(2,1);

if phase == 1
    % if contact is happened with can
    if grasping == 0
        if z(1) > x_can
            F_ext(1) = -k_can*(z(1) - x_can);    
        end
        if z(2) < y_table
            F_ext(2) = -k_table*(z(2) - y_table);
        end
    else 
        if z(2) < y_table
            F_ext(2) = -k_table*(z(2)-y_table);       
        else 
            if (abs(k_table*(z(2)-y_table)) < abs(mass_can*g))
                F_ext(2) = - k_table*(z(2)-y_table); 
            else 
                F_ext(2) = - mass_can*g;
            end    
        end
    end
elseif phase == 2
    if z(1) + l_can > x_wall 
        F_ext(1) = -k_wall*(z(1) + l_can -x_wall);
    end
    if z(2) < y_shelf
        F_ext(2) = -k_shelf*(z(2) - y_shelf);
    else 
        if (abs(k_shelf*(z(2)-y_shelf)) < abs(mass_can*g))
            F_ext(2) = - k_shelf*(z(2)-y_shelf); 
        else 
            F_ext(2) = - mass_can*g;
        end 
    end
else
    if z(1) + l_can > x_wall 
        F_ext(1) = -k_wall*(z(1) + l_can -x_wall);
    end
    if z(2) < y_shelf
        F_ext(2) = -k_shelf*(z(2) - y_shelf);
    end
end

== matlab function Tasks_union_3/TRAJECTORY/INTERPOLATOR ==
  data: xi input; z_des output; xf input; tf input; t input; v input; alpha input; dz_des output; ddz_des output
function [z_des, dz_des, ddz_des] = fcn(xi, xf, tf, t, v, alpha)

ta = alpha*tf; 
xa = (1/2)*v*ta;

if t >= 0 && t < ta
    ddz_des = v./ta;
    dz_des = ddz_des*t;
    z_des = xi + (1/2)*ddz_des*t^2;
elseif t >= ta && t < (tf-ta)
    ddz_des = [0; 0]; 
    dz_des = v; 
    z_des = xi + xa + dz_des*(t-ta);
elseif t >= (tf- ta) && t < tf
    ddz_des = -v./ta;
    dz_des = v + ddz_des*(t - (tf-ta));
    z_des = xi + xa + v*(tf-2*ta) + v*(t-(tf-ta)) + (1/2)*ddz_des*(t-(tf-ta))^2;
else 
    ddz_des = [0; 0];
    dz_des = [0; 0];
    z_des = xf;
end

end

== matlab function Tasks_union_3/MATLAB Function2 ==
  data: grasping input; phase input; K output; D output; M parameter; z input
function [K,D] = fcn(grasping,phase,M,z)
k1 = 200;
k2 = 200;
if phase == 1
    if grasping == 0
      k1 = 20;
      k2 = 20;
    else
      if z(2) > 0.1
       k1 = 200;
       k2 = 490.5; 
      else
       k1 = 20;
       k2 = 20;
      end
    end
elseif phase == 2
     k1 = 200;
     k2 = 490.5;
      if z(2) < 0.6
        k2 = 20;
      end 
      if z(1) > 1.3
        k1 = 20;
      end 
elseif phase == 3
     k1 = 20;
     k2 = 20;
end
K = [k1 0; 0 k2];
D = [sqrt(4*M*k1) 0; 0 sqrt(4*M*k2)];
end

== matlab function Tasks_union_3/RR_Model_Joint_Space/CORIOLIS ==
  data: q input size=2; Fc output double size=2; q_dot input size=2; a parameter; ac parameter; grasping input
function Fc = fcn(q,q_dot,a, ac, grasping)

C = zeros(2,2);
C = [-a*sin(q(2))*q_dot(2), -a*sin(q(2))*q_dot(1)-a*sin(q(2)*q_dot(2)); ...
    a*sin(q(2))*q_dot(1), 0];
% if grasping == 1
%     Cc = [-ac*sin(q(2))*q_dot(2), -ac*sin(q(2))*q_dot(1)-ac*sin(q(2)*q_dot(2)); ...
%           ac*sin(q(2))*q_dot(1), 0];
%       C =  C + Cc;
% end

Fc = C*q_dot;

end

== matlab function Tasks_union_3/M_D_S5/DAMPER ==
  data: dx input; y output; D input
function y = fcn(dx, D)
y = - D*dx;
end

== matlab function Tasks_union_3/M_D_S5/MASS^-1 ==
  data: M input; ddx output; F_tot input
function ddx = fcn(M,F_tot)
ddx = (M^-1)*F_tot;
end

== matlab function Tasks_union_3/M_D_S5/SPRING ==
  data: x input; tau output; K input
function tau = fcn(x, K)
tau= -K*x;
end

== matlab function Tasks_union_3/M_D_S3/DAMPER ==
  data: dx input; y output; D input
function y = fcn(dx, D)
y = - D*dx;
end

== matlab function Tasks_union_3/M_D_S3/MASS^-1 ==
  data: M input; ddx output; F_tot input
function ddx = fcn(M,F_tot)
ddx = (M^-1)*F_tot;
end

== matlab function Tasks_union_3/M_D_S3/SPRING ==
  data: x input; tau output; K input
function tau = fcn(x, K)
tau= -K*x;
end

== matlab function Tasks_union_3/F_ext1 ==
  data: z input; F_ext output; grasping input; mass_can parameter; g parameter; phase input; x_can parameter; y_table parameter; k_can parameter; k_table parameter; l_can parameter; x_wall parameter; y_shelf parameter; k_wall parameter; k_shelf parameter
function F_ext = fcn(z, grasping, mass_can, g, phase, x_can, y_table, k_can, k_table, l_can, x_wall, y_shelf, k_wall, k_shelf) 

% hypothesis: table reaction force with elastic behaviour
F_ext = zeros(2,1);

if phase == 1
    % if contact is happened with can
    if grasping == 0
        if z(1) > x_can
            F_ext(1) = -k_can*(z(1) - x_can);    
        end
        if z(2) < y_table
            F_ext(2) = -k_table*(z(2) - y_table);
        end
    else 
        if z(2) < y_table
            F_ext(2) = -k_table*(z(2)-y_table);       
        else 
            if (abs(k_table*(z(2)-y_table)) < abs(mass_can*g))
                F_ext(2) = - k_table*(z(2)-y_table); 
            else 
                F_ext(2) = - mass_can*g;
            end    
        end
    end
elseif phase == 2
    if z(1) + l_can > x_wall 
        F_ext(1) = -k_wall*(z(1) + l_can -x_wall);
    end
    if z(2) < y_shelf
        F_ext(2) = -k_shelf*(z(2) - y_shelf);
    else 
        if (abs(k_shelf*(z(2)-y_shelf)) < abs(mass_can*g))
            F_ext(2) = - k_shelf*(z(2)-y_shelf); 
        else 
            F_ext(2) = - mass_can*g;
        end 
    end
else
    if z(1) + l_can > x_wall 
        F_ext(1) = -k_wall*(z(1) + l_can -x_wall);
    end
    if z(2) < y_shelf
        F_ext(2) = -k_shelf*(z(2) - y_shelf);
    end
end

== matlab function Tasks_union_3/RR_Model_Joint_Space/GRAVITY ==
  data: q input size=2; G output double size=2; g parameter; l1 parameter; l2 parameter; m1 parameter; m2 parameter
function G = fcn(q,g, l1, l2, m1, m2)


G = [-(l1/2)*cos(q(1))*m1*g - m2*g*(l1*cos(q(1))+(l2/2)*cos(q(1)+q(2))); ...
    -m2*g*(l2/2)*cos(q(1)+q(2))];

end

== matlab function Tasks_union_3/RR_Model_Joint_Space/MASS^-1 ==
  data: q input size=2; ddq output size=2; F_tot input double size=2; I1 parameter; I2 parameter; l1 parameter; l2 parameter; m1 parameter; m2 parameter; grasping input; Ic parameter; mass_can parameter
function ddq = fcn(q,F_tot,I1, I2, l1, l2, m1, m2, grasping, Ic, mass_can)

mc = mass_can;

B = [((l1^2)/4)*m1 + I1 + m2*(l1^2) + m2*((l2^2)/4) + m2*l1*l2*cos(q(2)) + I2, m2*(((l1*l2)/2)*cos(q(2)) + (l2^2)/4) + I2; ...
    m2*(((l1*l2)/2)*cos(q(2)) + (l2^2)/4) + I2, m2*(l2^2)/4 + I2];

% if grasping == 1
%     Bc = [mc*((l1^2) + (l2^2) +2*l1*l2*cos(q(2))) + Ic, mc*((l2^2) + l1*l2*cos(q(2))) + Ic; ...
%           mc*((l2^2) + l1*l2*cos(q(2))) + Ic, mc*(l2^2)+ Ic];
%     B = B + Bc;
% end

ddq = B\F_tot;                      % Ftot*M^-1

end

== matlab function Tasks_union_3/RR_Model_Joint_Space/MATLAB Function ==
  data: F input size=2; F_ext output double size=2; q input size=2; l1 parameter; l2 parameter
function F_ext = fcn(F,q,l1, l2)


Ja = [-l1*sin(q(1)) - l2*sin(q(1)+q(2)), -l2*sin(q(1)+q(2)); ...
    l1*cos(q(1)) + l2*cos(q(1)+q(2)), l2*cos(q(1)+q(2))];

F_ext = Ja'*F;

end
